simulink model "my_demo"  (R2012b)
settings: Solver=FixedStepDiscrete  StartTime=0.0  StopTime=Inf  FixedStep=0.033  RelTol=1e-3
values from neighbouring files (symbols this model uses):
  A = 0.1    [param.m]
  inc = 0.05    [param.m]
  UMAX = 10    [param.m]
  XG = 1    [param.m]
  YG = 1    [param.m]
undefined symbols (not defined in the file or in its folder): LF, magnitude, serial
libraries: instrumentlib x3, simulink x1, vrlib x1, simiam x1
settings Model: Creator=jdelacroix  LastModifiedBy=samati
settings DataIOCC: SignalLoggingSaveFormat=ModelDataLogs  SaveOutput=off  SaveTime=off
settings DebuggingCC: MultiTaskDSMMsg=warning  MultiTaskCondExecSysMsg=none  FcnCallInpInsideContextMsg=EnableAllAsWarning  StrictBusMsg=None
settings RTWCC: IncludeERTFirstTime=on
settings CodeAppCC: CustomSymbolStrType=$N$R$M_T  InternalIdentifier=Shortened
settings GRTTargetCC: CodeReplacementLibrary=None  CPPClassGenCompliant=on

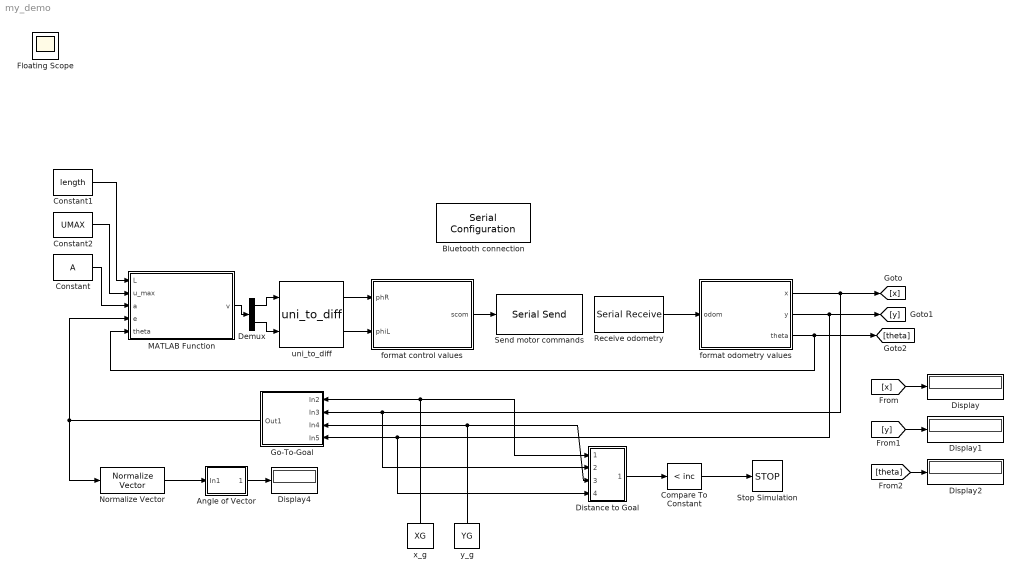
== system my_demo ==
  Angle of Vector : Subsystem
      mask Display:
      | port_label('input', 1, 'u')
      | port_label('output', 1, 'theta')
  Bluetooth connection : instrumentlib/Serial Configuration  Priority=-200000  ComPortMenu=COM1  ComPort=COM1  ObjConstructor=serial('COM1');  BaudRate=9600  DataBits=8  Parity=none  StopBits=1  FlowControl=none  Timeout=10  ByteOrder=LittleEndian
  Compare To Constant : simulink/Logic and Bit Operations/Compare To Constant  relop=<  const=inc  OutDataTypeStr=boolean
  Constant : Constant  Value=A
  Constant1 : Constant  Value=length
  Constant2 : Constant  Value=UMAX
  Demux : Demux  Outputs=2
  Display{,1..2,4} (4 alike) : Display
  Distance to Goal : Subsystem
      mask Display:
      | port_label('input', 1, 'x_g')
      | port_label('input', 2, 'x')
      | port_label('input', 3, 'y_g')
      | port_label('input', 4, 'y')
      | port_label('output', 1, 'd')
  Go-To-Goal : Subsystem
      mask Display:
      | port_label('input', 1, 'x_g')
      | port_label('input', 2, 'x')
      | port_label('input', 3, 'y_g')
      | port_label('input', 4, 'y')
      | port_label('output', 1, 'u_gtg')
  MATLAB Function : MATLAB Function  TreatAsAtomicUnit=on
  Normalize Vector : vrlib/Utilities/Normalize Vector  maxzero=0
  Receive odometry : instrumentlib/Serial Receive  ComPortMenu=COM1  ComPort=COM1  ObjConstructor=serial('COM1');  Terminator=<none>  DataSize=[1 1]  DataType=uint8  EnableBlockingMode=on  ActionDataUnavailable=Output last received value  CustomValue=0  SampleTime=0.01
  Send motor commands : instrumentlib/Serial Send  ComPortMenu=COM1  ComPort=COM1  ObjConstructor=serial('COM1');  Terminator=LF ('\n')  EnableBlockingMode=on
  Stop Simulation : Stop
  format control values : MATLAB Function  TreatAsAtomicUnit=on
  format odometry values : MATLAB Function  TreatAsAtomicUnit=on
  uni_to_diff : simiam/uni_to_diff  wheel_radius=radius  wheel_base_length=length
  x_g : Constant  Value=XG
  y_g : Constant  Value=YG
  Floating Scope : Scope
  wires:
  uni_to_diff/1 -> format control values/1(phR)
  uni_to_diff/2 -> format control values/2(phiL)
  format odometry values/1(x) -> Distance to Goal/2(In2), Go-To-Goal/2(In3), [x]
  format odometry values/2(y) -> Distance to Goal/4(In4), Go-To-Goal/4(In5), [y]
  [theta] -> Display2/1
  [y] -> Display1/1
  [x] -> Display/1
  x_g/1 -> Go-To-Goal/1(In2), Distance to Goal/1(In1)
  y_g/1 -> Go-To-Goal/3(In4), Distance to Goal/3(In3)
  Go-To-Goal/1(Out1) -> Normalize Vector/1, MATLAB Function/4(e)
  format odometry values/3(theta) -> MATLAB Function/5(theta), [theta]
  Normalize Vector/1 -> Angle of Vector/1(In1)
  Angle of Vector/1(Out1) -> Display4/1
  Distance to Goal/1(Out1) -> Compare To Constant/1
  Compare To Constant/1 -> Stop Simulation/1
  Demux/1 -> uni_to_diff/1
  Demux/2 -> uni_to_diff/2
  MATLAB Function/1(v) -> Demux/1
  format control values/1(scom) -> Send motor commands/1
  Receive odometry/1 -> format odometry values/1(odom)
  Constant1/1 -> MATLAB Function/1(L)
  Constant/1 -> MATLAB Function/3(a)
  Constant2/1 -> MATLAB Function/2(u_max)

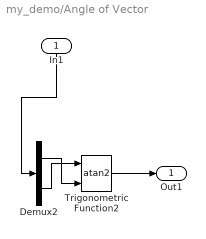
== system my_demo/Angle of Vector ==
  In1 : Inport
  Demux2 : Demux  Outputs=2
  Trigonometric Function2 : Trigonometry  Operator=atan2
  Out1 : Outport
  wires:
  Trigonometric Function2/1 -> Out1/1
  Demux2/1 -> Trigonometric Function2/2
  Demux2/2 -> Trigonometric Function2/1
  In1/1 -> Demux2/1

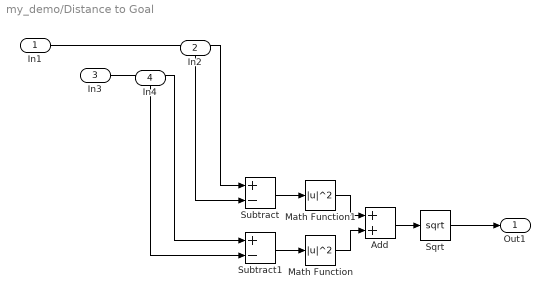
== system my_demo/Distance to Goal ==
  In1 : Inport
  In2 : Inport  Port=2
  In3 : Inport  Port=3
  In4 : Inport  Port=4
  Add : Sum
  Math Function : Math  Operator=magnitude^2  SaturateOnIntegerOverflow=on
  Math Function1 : Math  Operator=magnitude^2  SaturateOnIntegerOverflow=on
  Sqrt : Sqrt  SaturateOnIntegerOverflow=on
  Subtract : Sum  Inputs=+-
  Subtract1 : Sum  Inputs=+-
  Out1 : Outport
  wires:
  In4/1 -> Subtract1/2
  Subtract1/1 -> Math Function/1
  Math Function/1 -> Add/2
  Sqrt/1 -> Out1/1
  Subtract/1 -> Math Function1/1
  Math Function1/1 -> Add/1
  Add/1 -> Sqrt/1
  In2/1 -> Subtract/2
  In3/1 -> Subtract1/1
  In1/1 -> Subtract/1

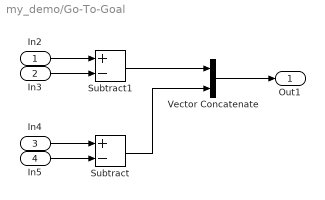
== system my_demo/Go-To-Goal ==
  In2 : Inport
  In3 : Inport  Port=2
  In4 : Inport  Port=3
  In5 : Inport  Port=4
  Subtract : Sum  Inputs=+-
  Subtract1 : Sum  Inputs=+-
  Vector Concatenate : Concatenate  Mode=Multidimensional array
  Out1 : Outport
  wires:
  In5/1 -> Subtract/2
  In2/1 -> Subtract1/1
  In3/1 -> Subtract1/2
  In4/1 -> Subtract/1
  Vector Concatenate/1 -> Out1/1
  Subtract1/1 -> Vector Concatenate/1
  Subtract/1 -> Vector Concatenate/2

== matlab function my_demo/format control values ==
  data: phR input; phiL input; scom output
function scom = fcontrol(phR, phiL)

% Find signs
if(phiL>=0) signL = '+';
else  signL = '';
end

if(phiR>=0) signR = '+';
else  signR = '';
end

% Create string needed to send commands to robot
scom = [signL, num2str(phiL), signR, num2str(phiR)];

end

== matlab function my_demo/MATLAB Function ==
  data: L input; u_max input; a input; e input; v output; theta input
function v = my_demo(L, u_max, a, e, theta)

mat = [1 0; 0 1/l];
R = [cos(-theta) -sin(-theta); sin(-theta) cos(-theta)];

k1 = 1./exp(abs(e(1))) + (u_max * (1-exp(-a.*e(1).^2))) ./ abs(e(1));
k2 = 1./exp(abs(e(2))) + (u_max * (1-exp(-a.*e(2).^2))) ./ abs(e(2));
K = [k1 0; 0 k2];

v = mat*R*K*e;

== matlab function my_demo/format odometry values ==
  data: x output; odom input; y output; theta output
function [x, y, theta] = fodom(odom)

x = 0;
y = 0;
theta = 0;

end
